simulink library "Window_Control"  (R2018b)
settings: Solver=ode45  StartTime=0.0  StopTime=10.0  RelTol=1e-3  EnableMultiTasking=on
libraries: simulink x4
settings Model: Creator=lena.frank  LastModifiedBy=P41573
settings DataIOCC: LimitDataPoints=on  SaveFormat=Array  SignalLoggingSaveFormat=ModelDataLogs
settings OptimizationCC: ExpressionDepthLimit=2147483647  LifeSpan=inf
settings DebuggingCC: UnderspecifiedInitializationDetection=Classic  MergeDetectMultiDrivingBlocksExec=none  SolverPrmCheckMsg=warning  FcnCallInpInsideContextMsg=warning  StateNameClashWarn=warning  SFUnexpectedBacktrackingDiag=warning  SFNoUnconditionalDefaultTransitionDiag=warning  SFExecutionAtInitializationDiag=none
settings HardwareCC: ProdBitPerPointer=32  ProdBitPerSizeT=32  ProdBitPerPtrDiffT=32  ProdLargestAtomicFloat=None  ProdIntDivRoundTo=Undefined  ProdEndianess=Unspecified  ProdWordSize=32  ProdHWDeviceType=32-bit Generic
settings ModelReferenceCC: PropagateSignalLabelsOutOfModel=off
settings SFSimCC: SimUseLocalCustomCode=off
settings RTWCC: RTWUseLocalCustomCode=off
settings CodeAppCC: StateflowObjectComments=on
settings GRTTargetCC: TargetLangStandard=C89/C90 (ANSI)  GeneratePreprocessorConditionals=Disable all  CombineOutputUpdateFcns=off  GRTInterface=on
settings ConfigComp: CovMetricSettings=dw  CovHtmlReporting=on  CovSaveCumulativeToWorkspaceVar=on  CovSaveSingleToWorkspaceVar=on  CovExternalEMLEnable=off

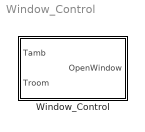
== system Window_Control ==
  Window_Control : Subsystem  mask(Window Control){Topen=24, Tclose=23, TrAboveTa=2, TaTooCold=12, timeFIR=24, TaIni=12, starttime=8, stoptime=22}
      mask prompts: Topen "Open window if Troom is above [°C]"; Tclose "Close window if Troom is below [°C]"; TrAboveTa "Open window if Troom is above Tamb [K]"; TaTooCold "Close window if Tamb is below [°C]"; timeFIR "Average time for Tamb in h (only integer values)"; TaIni "Initial value for Tamb in °C"; starttime "Start time in the morning [h]"; stoptime "Stop time in the evening [h]"
      mask help:
      | Control for free driven passive cooling realized by tilted windows.
      | Window is opened if:
      | + Room temperature (Troom) is above a fixed value
      | + Outdoor ambient temperature (Tamb) is below Troom
      | + Average of Tamb is not too cold
      | + During the day (starttime <= time < stoptime)
      mask Help: web(fullfile(path_carnot('help'),'Window_Control.html'),'-helpbrowser')
      mask TypeOptions Topen: RelayTroom/OnSwitchValue
      mask TypeOptions Tclose: RelayTroom/OffSwitchValue
      mask TypeOptions TrAboveTa: Troom_GE_Tamb/const
      mask TypeOptions TaTooCold: Tamb_GT_Const/const
      mask TypeOptions TaIni: MovingAverage/InitialStates
      mask TypeOptions starttime: FromMorning/const
      mask TypeOptions stoptime: TillEvening/const
      mask Display:
      | plot(-5,10,90,80,[20 70 70 20 20],[20 20 70 70 20],...
      |     [20 70 80 30 20],[20 20 65 65 20])

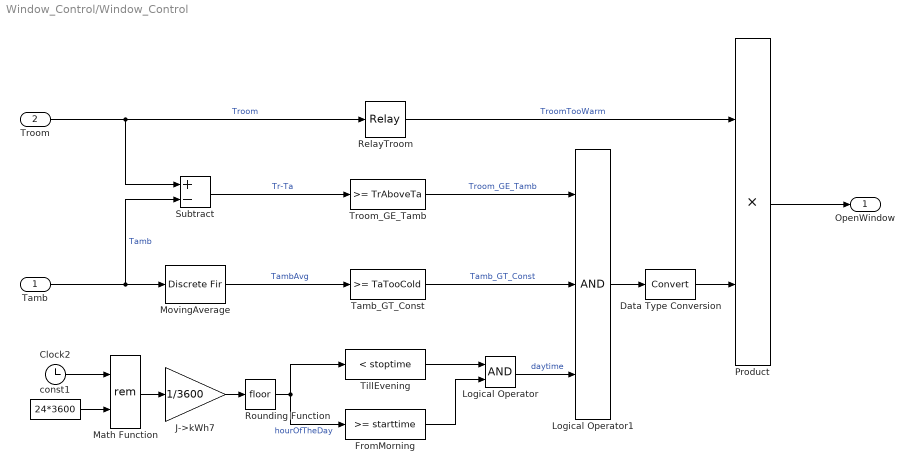
== system Window_Control/Window_Control ==
  Tamb : Inport
  Troom : Inport  Port=2
  Clock2 : Clock
  Data Type Conversion : DataTypeConversion
  FromMorning : simulink/Logic and Bit Operations/Compare To Constant  relop=>=  const=starttime  OutDataTypeStr=boolean
  J->kWh7 : Gain  Gain=1/3600  SaturateOnIntegerOverflow=on  OutDataTypeStr=Inherit: Same as input  ParamDataTypeStr=Inherit: Same as input
  Logical Operator : Logic  AllPortsSameDT=off  OutDataTypeStr=boolean
  Logical Operator1 : Logic  Inputs=3  AllPortsSameDT=off  OutDataTypeStr=boolean
  Math Function : Math  Operator=rem  SaturateOnIntegerOverflow=on
  MovingAverage : DiscreteFir  Coefficients=ones(1,floor(timeFIR))*(1/floor(timeFIR))  InitialStates=TaIni  SampleTime=3600  AccumDataTypeStr=Inherit: Same as product output  RndMeth=Nearest
  Product : Product  RndMeth=Zero
  RelayTroom : Relay  OnSwitchValue=Topen  OffSwitchValue=Tclose
  Rounding Function : Rounding
  Subtract : Sum  Inputs=+-
  Tamb_GT_Const : simulink/Logic and Bit Operations/Compare To Constant  relop=>=  const=TaTooCold  OutDataTypeStr=boolean
  TillEvening : simulink/Logic and Bit Operations/Compare To Constant  relop=<  const=stoptime  OutDataTypeStr=boolean
  Troom_GE_Tamb : simulink/Logic and Bit Operations/Compare To Constant  relop=>=  const=TrAboveTa  OutDataTypeStr=boolean
  const1 : Constant  Value=24*3600
  OpenWindow : Outport
  wires:
  MovingAverage/1 -> Tamb_GT_Const/1  "TambAvg"
  RelayTroom/1 -> Product/1  "TroomTooWarm"
  Product/1 -> OpenWindow/1
  Data Type Conversion/1 -> Product/2
  Tamb_GT_Const/1 -> Logical Operator1/2  "Tamb_GT_Const"
  Logical Operator1/1 -> Data Type Conversion/1
  Troom_GE_Tamb/1 -> Logical Operator1/1  "Troom_GE_Tamb"
  Subtract/1 -> Troom_GE_Tamb/1  "Tr-Ta"
  Troom/1 -> RelayTroom/1, Subtract/1  "Troom"
  Logical Operator/1 -> Logical Operator1/3  "daytime"
  Tamb/1 -> MovingAverage/1, Subtract/2  "Tamb"
  FromMorning/1 -> Logical Operator/2
  TillEvening/1 -> Logical Operator/1
  Rounding Function/1 -> FromMorning/1, TillEvening/1  "hourOfTheDay"
  J->kWh7/1 -> Rounding Function/1
  Math Function/1 -> J->kWh7/1
  const1/1 -> Math Function/2
  Clock2/1 -> Math Function/1
